simulink model "Test_HPC"  (R2025b)
settings: Solver=VariableStepAuto  StartTime=0.0  StopTime=inf  RelTol=1e-3
libraries: TCU_HPC x1
settings Model: Creator=joshu  LastModifiedBy=joshu

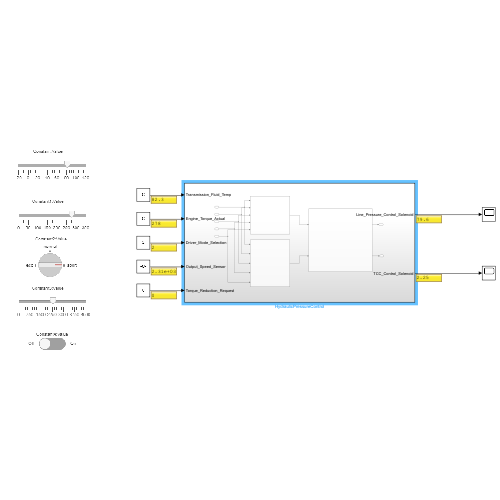
[thumbnail: Simulink's stored preview of the top-level diagram]
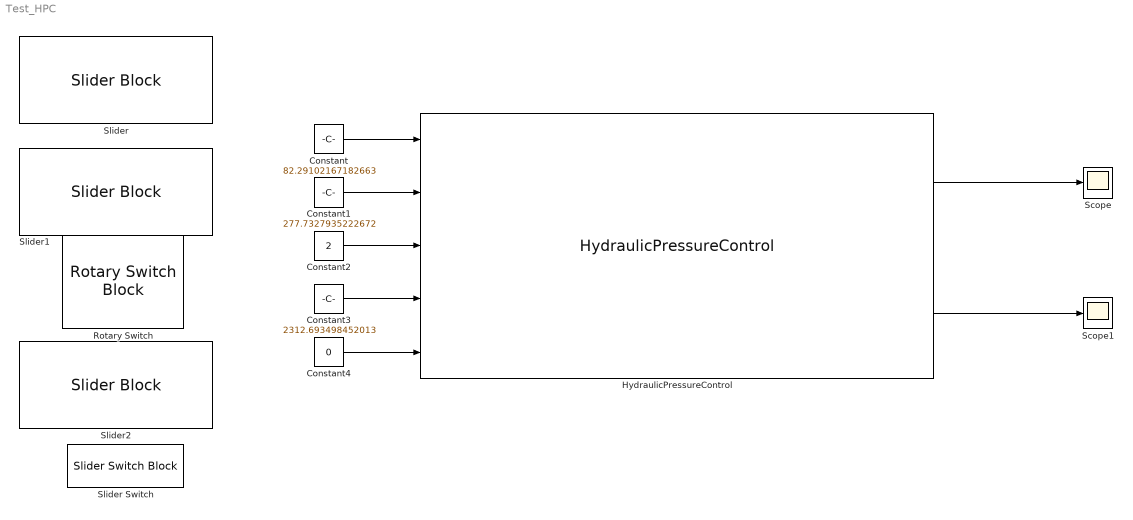
== system Test_HPC ==
  Constant : Constant  Value=82.29102167182663
  Constant1 : Constant  Value=277.7327935222672
  Constant2 : Constant  Value=2
  Constant3 : Constant  Value=2312.693498452013
  Constant4 : Constant  Value=0
  HydraulicPressureControl : TCU_HPC/HydraulicPressureControl  SystemSampleTime=-1  VariantActivationTime=update diagram  EmptyChoice=off  PassThrough=off  PassThroughVariantControl=(default)  EmptyChoiceVariantControl=(default)  AllowFlexibleInterface=on  Latency=0  AutoFrameSizeCalculation=off
  Rotary Switch : RotarySwitchBlock
  Scope : Scope
  Scope1 : Scope
  Slider : SliderBlock  ScaleMin=-20  ScaleMax=120  TickInterval=20
  Slider Switch : SliderSwitchBlock
  Slider1 : SliderBlock  ScaleMax=350  TickInterval=50
  Slider2 : SliderBlock  ScaleMax=4500
  wires:
  Constant/1 -> HydraulicPressureControl/1
  Constant1/1 -> HydraulicPressureControl/2
  Constant2/1 -> HydraulicPressureControl/3
  Constant3/1 -> HydraulicPressureControl/4
  Constant4/1 -> HydraulicPressureControl/5
  HydraulicPressureControl/1 -> Scope/1
  HydraulicPressureControl/2 -> Scope1/1
